simulink model "zhh2"  (Simulink 8.3)
settings: Solver=FixedStepDiscrete  StartTime=0.0  StopTime=inf  MaxStep=1/256  RelTol=1e-3
model workspace (MAT data in the model file):
  device_serial = 'HA-2012.04.03'
  sample_rate = 256
  buffer_size = 8
  number_of_channels = 18
  cfg_native : struct (value not decoded)
undefined symbols (not defined in the file or in its folder): HA
libraries: gHIampTools x2, ScopeScaler x1, gHIampLib x1, gtecHighspeedLib x1
settings Model: Creator=gtec  LastModifiedBy=dell
settings OptimizationCC: ExpressionDepthLimit=2147483647  InitFltsAndDblsToZero=on
settings DebuggingCC: MultiTaskCondExecSysMsg=none  FcnCallInpInsideContextMsg=EnableAllAsWarning

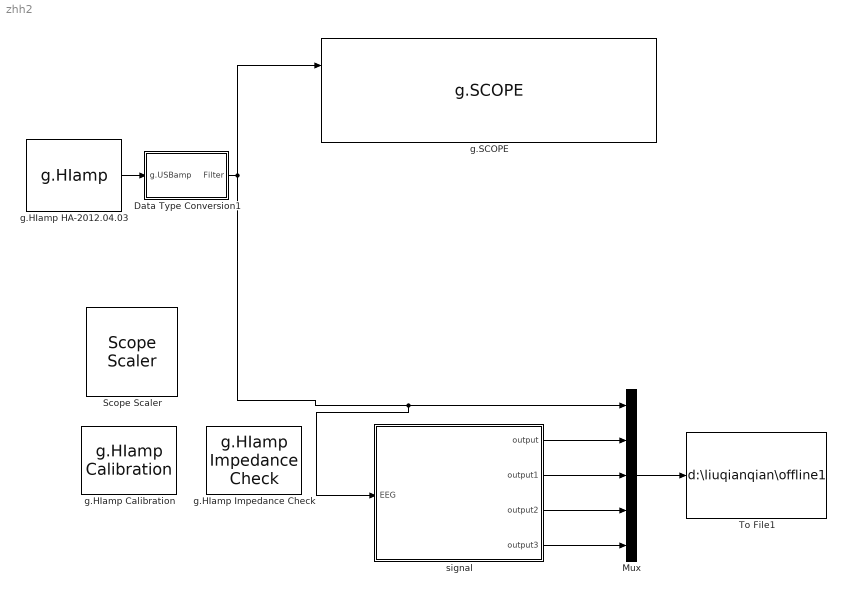
== system zhh2 ==
  Data Type Conversion1 : Subsystem
  Mux : Mux  Inputs=5
  Scope Scaler : ScopeScaler/Scope Scaler  SystemSampleTime=-1
  To File1 : ToFile  Filename=d:\liuqianqian\offline1  MatrixName=y
  g.HIamp Calibration : gHIampTools/g.HIamp Calibration
  g.HIamp HA-2012.04.03 : gHIampLib/g.HIamp  sample_rate=256  buffer_size=8  number_of_channels=18  device_serial=HA-2012.04.03
  g.HIamp Impedance Check : gHIampTools/g.HIamp Impedance Check
  g.SCOPE : gtecHighspeedLib/g.SCOPE
  signal : Subsystem  mask{host='192.168.1.4;192.168.1.2', socket='50000;31500', NumCustomCmds=12, ISI=200, SimNumTrials=20, ResetSpellerPeriod=300, PausePeriod=500, SampleRate=256, Determination=1, channels=16, selectchannles=[2:17], BaseAver=1, rep=2, targetp=[1 2 3 4 5 99 99 99 14 15 16 17 18 99 99 99 31 32 33 34 35 99 99 99 99 99  ], starget=4, traintime=4}
      mask prompts: host "P300host"; socket "P300socket"; NumCustomCmds "P300NumCustomCmds"; ISI "P300ISI"; SimNumTrials "P300SimNumTrials"; ResetSpellerPeriod "P300ResetSpellerPeriod"; PausePeriod "P300PausePeriod"; SampleRate "P300SampleRate"; Determination "P300Determination(classfier,yes,no)"; channels "Channles"; selectchannles "select Channels"; BaseAver "P300BaseAverage"; rep "P300reptimes"; targetp "P300target"; starget "s-target"
      mask Display:
      | image(imread('D:\vep_competition\bci.png'))
      | port_label('output', 1, 'flash')
      | port_label('output', 2, 'trial')
      | port_label('input', 1, 'EEG')
  wires:
  Mux/1 -> To File1/1
  signal/1(output) -> Mux/2
  signal/2(output1) -> Mux/3
  signal/3(output2) -> Mux/4
  signal/4(output3) -> Mux/5
  g.HIamp HA-2012.04.03/1 -> Data Type Conversion1/1(g.USBamp)
  Data Type Conversion1/1(Filter) -> Mux/1, signal/1(EEG), g.SCOPE/1

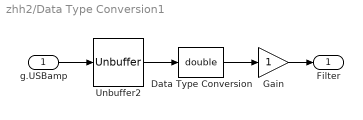
== system zhh2/Data Type Conversion1 ==
  g.USBamp : Inport  Priority=1
  Data Type Conversion : DataTypeConversion  OutDataTypeStr=double
  Gain : Gain  SampleTime=1/256  SaturateOnIntegerOverflow=on  OutDataTypeStr=Inherit: Same as input  ParamDataTypeStr=Inherit: Same as input
  Unbuffer2 : Unbuffer
  Filter : Outport
  wires:
  Data Type Conversion/1 -> Gain/1
  Unbuffer2/1 -> Data Type Conversion/1
  Gain/1 -> Filter/1
  g.USBamp/1 -> Unbuffer2/1

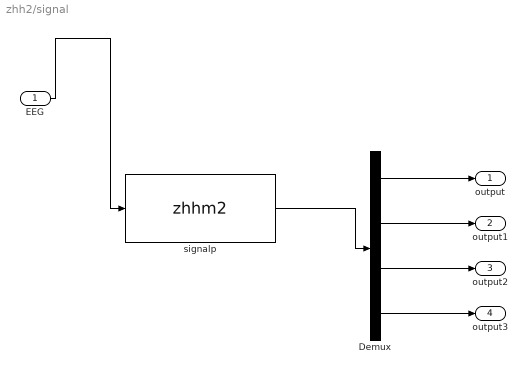
== system zhh2/signal ==
  EEG : Inport
  Demux : Demux
  signalp : S-Function  FunctionName=zhhm2  Parameters=host,socket,NumCustomCmds,ISI,SimNumTrials,ResetSpellerPeriod,PausePeriod,SampleRate,Determination,channels,selectchannles,BaseAver,rep,targetp,starget,traintime  EnableBusSupport=off
  output : Outport
  output1 : Outport  Port=2
  output2 : Outport  Port=3
  output3 : Outport  Port=4
  wires:
  EEG/1 -> signalp/1
  signalp/1 -> Demux/1
  Demux/1 -> output/1
  Demux/2 -> output1/1
  Demux/3 -> output2/1
  Demux/4 -> output3/1
